simulink model "combining_trajectory_parking_pietro"  (R2025b)
settings: Solver=ode5  StartTime=0.0  StopTime=25  FixedStep=0.0001  MaxStep=0.01  RelTol=1e-3
values from neighbouring files (symbols this model uses):
  ang_velocity = 3    [traj.m]
  speed = 15    [traj.m]
  time_vec_circ = time_vec_circ'    [traj.m]
  waypoints = [ ... (first row only)    [traj.m]
libraries: dspsigops x3
settings Model: Creator=Cris  LastModifiedBy=pietr
settings DebuggingCC: UnderspecifiedInitializationDetection=Classic  MergeDetectMultiDrivingBlocksExec=none
settings ModelReferenceCC: PropagateSignalLabelsOutOfModel=off

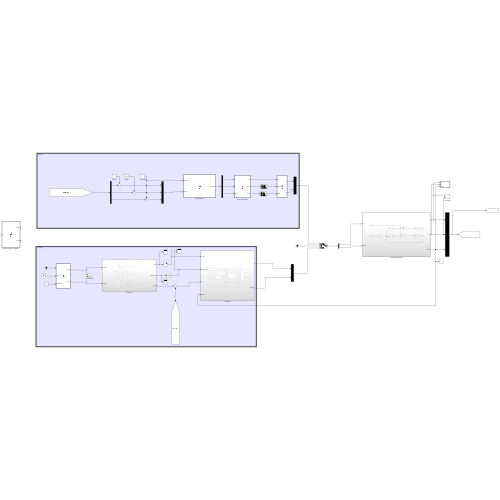
[thumbnail: Simulink's stored preview of the top-level diagram]
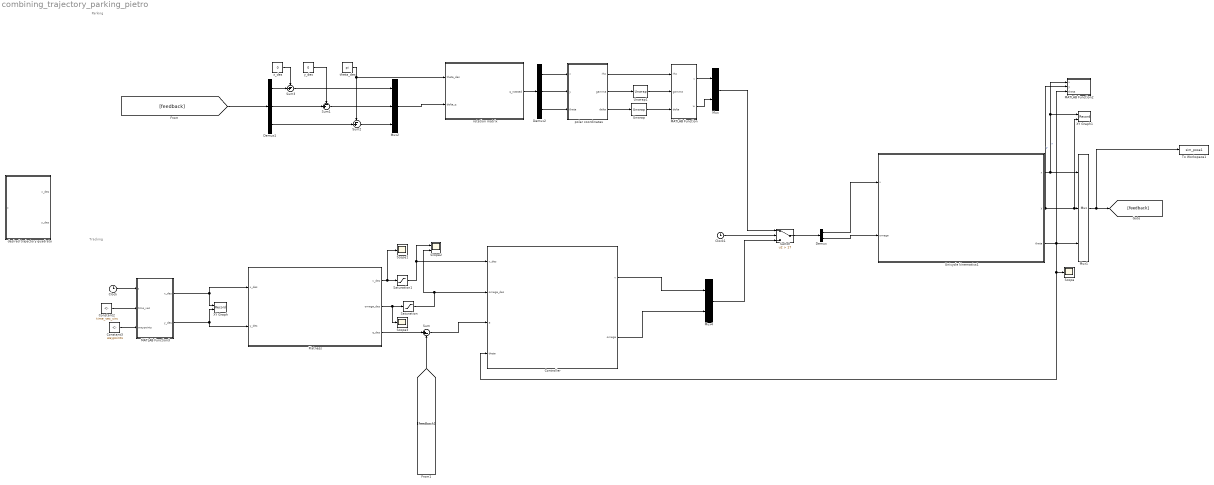
== system combining_trajectory_parking_pietro ==
  note: Tracking
  note: Parking
  Clock : Clock
  Clock1 : Clock
  Constant2 : Constant  Value=time_vec_circ
  Constant3 : Constant  Value=waypoints
  Controller : Subsystem
  Demux : Demux  Outputs=2
  Demux1 : Demux  Outputs=3
  Demux2 : Demux  Outputs=3
  Flatness : Subsystem
  MATLAB Function : MATLAB Function  TreatAsAtomicUnit=on
  MATLAB Function2 : MATLAB Function  TreatAsAtomicUnit=on
  MATLAB Function3 : MATLAB Function  TreatAsAtomicUnit=on
  Mux : Mux  Inputs=2
  Mux1 : Mux  Inputs=3
  Mux2 : Mux  Inputs=3
  Mux4 : Mux  Inputs=2
  Saturation : Saturate  UpperLimit=ang_velocity  LowerLimit=-ang_velocity
  Saturation1 : Saturate  UpperLimit=speed  LowerLimit=-speed
  Scope : Scope
      settings: ActiveDisplayYMinimum=-2.2678628072381004  ActiveDisplayYMaximum=10.713846589075981
  Scope1 : Scope
      settings: ActiveDisplayYMinimum=-58.541647894510909  ActiveDisplayYMaximum=33.790255014407059  DataLoggingVariableName=ScopeData3
  Scope2 : Scope  NumInputPorts=2
      settings: ActiveDisplayYMinimum=0.14603727460674376  ActiveDisplayYMaximum=5.9509475084943659
  Scope3 : Scope
      settings: ActiveDisplayYMinimum=-7.9417132034456789E+8  ActiveDisplayYMaximum=7.1473011331260653E+9  DataLoggingVariableName=ScopeData4
  Sum : Sum  Inputs=|+-
  Sum1 : Sum  Inputs=-+|
  Sum2 : Sum  Inputs=-+|
  Sum3 : Sum  Inputs=-+|
  Switch : Switch  Criteria=u2 > Threshold  Threshold=17  SaturateOnIntegerOverflow=off  InputSameDT=off
  To Workspace1 : ToWorkspace  VariableName=sim_pose1  SaveFormat=Timeseries  SampleTime=-1
  Unicycle kinematics1 : Subsystem
  Unwrap : dspsigops/Unwrap  tol=pi  InputProcessing=Columns as channels (frame based)  running=off
  Unwrap1 : dspsigops/Unwrap  tol=pi  InputProcessing=Columns as channels (frame based)  running=off
  XY Graph : Record  NumPorts=2.0  FileSettingsInternal="{\"entries\":[{\"content\":{\"excelSettings\":{\"content\":{},\"type\":\"Streamout.ExcelSettings\"},\"parquetSettings\":{\"content\":{},\"type\":\"Streamout.ParquetSettings\"}},\"type\":\"Streamout.FileSettingStorage\",\"uuid\":\"\"}],\"packageUris\":[\"http:\\/\\/schema.mathworks.com\\/mf0\\/streamout_blocks\\/R2020a\"],\"version\":\"1.0\"}"  FrameSettings=[0, 0]  Layout=[1 1]  SignalsInternal="{\"entries\":[{\"content\":{\"signals\":[{\"content\":{\"blockPath\":[],\"dimensions\":[1],\"domain\":\"\",\"lineColor\":\"#a2142f\",\"plots\":[ 1 ],\"port\":1,\"sid\":[\"\"],\"signalID\":1,\"signalName\":\"MATLAB Function3:1\"},\"type\":\"RecordBlkView.Signal\",\"uuid\":\"\"},{\"content\":{\"blockPath\":[],\"dimensions\":[1],\"domain\":\"\",\"lineColor\":\"#139fff\",\"plots\":[ 1 ],\"port\":2,\"sid\":[\"\"],\"signalID\":2,\"signalName\":\"MATLAB Function3:2\"},\"type\":\"RecordBlkView.Signal\",\"uuid\":\"\"}]},\"type\":\"RecordBlkView.InputSignals\",\"uuid\":\"\"}],\"packageUris\":[\"http:\\/\\/schema.mathworks.com\\/mf0\\/streamout_blocks\\/R2020a\"],\"version\":\"1.0\"}"  VisualizationBindings="{\"xyplotplugin\":{\"info\":[{\"series\":[{\"bindingParametersList\":[{\"parameter\":\"X-Axis\",\"signalID\":1,\"signalName\":\"MATLAB Function3:1\"},{\"parameter\":\"Y-Axis\",\"signalID\":2,\"signalName\":\"MATLAB Function3:2\"}],\"seriesID\":0}],\"subplotID\":1}]}}"  CompatibilityTag=XY
  XY Graph1 : Record  NumPorts=2.0  FileSettingsInternal="{\"entries\":[{\"content\":{\"excelSettings\":{\"content\":{},\"type\":\"Streamout.ExcelSettings\"},\"parquetSettings\":{\"content\":{},\"type\":\"Streamout.ParquetSettings\"}},\"type\":\"Streamout.FileSettingStorage\",\"uuid\":\"\"}],\"packageUris\":[\"http:\\/\\/schema.mathworks.com\\/mf0\\/streamout_blocks\\/R2020a\"],\"version\":\"1.0\"}"  FrameSettings=[0, 0]  Layout=[1 1]  SignalsInternal="{\"entries\":[{\"content\":{\"signals\":[{\"content\":{\"blockPath\":[],\"dimensions\":[1],\"domain\":\"\",\"lineColor\":\"#a2142f\",\"plots\":[ 1 ],\"port\":1,\"sid\":[\"\"],\"signalID\":1,\"signalName\":\"x\"},\"type\":\"RecordBlkView.Signal\",\"uuid\":\"\"},{\"content\":{\"blockPath\":[],\"dimensions\":[1],\"domain\":\"\",\"lineColor\":\"#139fff\",\"plots\":[ 1 ],\"port\":2,\"sid\":[\"\"],\"signalID\":2,\"signalName\":\"y\"},\"type\":\"RecordBlkView.Signal\",\"uuid\":\"\"}]},\"type\":\"RecordBlkView.InputSignals\",\"uuid\":\"\"}],\"packageUris\":[\"http:\\/\\/schema.mathworks.com\\/mf0\\/streamout_blocks\\/R2020a\"],\"version\":\"1.0\"}"  VisualizationBindings="{\"xyplotplugin\":{\"info\":[{\"series\":[{\"bindingParametersList\":[{\"parameter\":\"X-Axis\",\"signalID\":1,\"signalName\":\"x\"},{\"parameter\":\"Y-Axis\",\"signalID\":2,\"signalName\":\"y\"}],\"seriesID\":0}],\"subplotID\":1}]}}"  CompatibilityTag=XY
  desired trajectory quadrato : MATLAB Function  TreatAsAtomicUnit=on
  polar coordinates : MATLAB Function  TreatAsAtomicUnit=on
  rotation matrix : MATLAB Function  TreatAsAtomicUnit=on
  theta_des : Constant  Value=pi
  x_des : Constant  Value=0
  y_des : Constant  Value=0
  wires:
  Flatness/3(q_des) -> Sum/1
  Controller/2(omega) -> Mux4/2
  Demux1/3 -> Sum2/2
  theta_des/1 -> Sum2/1, rotation matrix/1(theta_des)
  rotation matrix/1(q_rotated) -> Demux2/1
  Sum1/1 -> Mux2/2
  Unwrap/1 -> MATLAB Function/3(delta)
  Sum2/1 -> Mux2/3
  y_des/1 -> Sum1/1
  x_des/1 -> Sum3/1
  Demux2/1 -> polar coordinates/1(x)
  Mux1/1 -> [feedback], To Workspace1/1
  Mux2/1 -> rotation matrix/2(delta_q)
  Demux2/3 -> polar coordinates/3(theta)
  Unicycle kinematics1/2(y) -> MATLAB Function2/2(y), XY Graph1/2, Mux1/2  "y"
  Unicycle kinematics1/1(x) -> MATLAB Function2/1(x), XY Graph1/1, Mux1/1  "x"
  Unwrap1/1 -> MATLAB Function/2(gamma)
  Sum3/1 -> Mux2/1
  Unicycle kinematics1/3(theta) -> Controller/4(theta), Scope/1, Mux1/3, MATLAB Function2/3(theta)
  polar coordinates/3(delta) -> Unwrap/1
  polar coordinates/2(gamma) -> Unwrap1/1
  Demux1/2 -> Sum1/2
  Demux1/1 -> Sum3/2
  Demux2/2 -> polar coordinates/2(y)
  polar coordinates/1(rho) -> MATLAB Function/1(rho)
  Clock1/1 -> Switch/2
  [feedback] -> Demux1/1
  [feedback] -> Sum/2
  MATLAB Function/1(v) -> Mux/1
  MATLAB Function/2(w) -> Mux/2
  Demux/1 -> Unicycle kinematics1/1(v)
  Demux/2 -> Unicycle kinematics1/2(omega)
  Controller/1(v) -> Mux4/1
  Mux/1 -> Switch/1
  Switch/1 -> Demux/1
  Mux4/1 -> Switch/3
  Constant3/1 -> MATLAB Function3/3(waypoints)
  MATLAB Function3/1(x_des) -> Flatness/1(x_des), XY Graph/1
  MATLAB Function3/2(y_des) -> XY Graph/2, Flatness/2(y_des)
  Flatness/2(omega_des) -> Scope3/1, Saturation/1
  Saturation/1 -> Scope2/2, Controller/2(omega_des)
  Flatness/1(v_des) -> Saturation1/1, Scope1/1
  Saturation1/1 -> Controller/1(v_des), Scope2/1
  Sum/1 -> Controller/3(e)
  Clock/1 -> MATLAB Function3/1(t)
  Constant2/1 -> MATLAB Function3/2(time_vec)

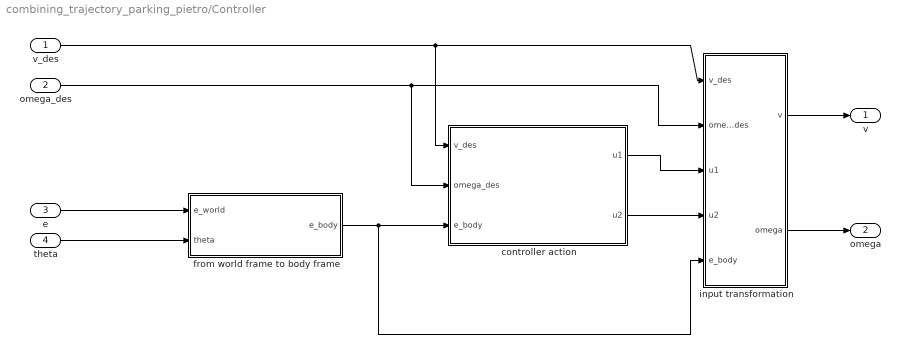
== system combining_trajectory_parking_pietro/Controller ==
  v_des : Inport
  omega_des : Inport  Port=2
  e : Inport  Port=3
  theta : Inport  Port=4
  controller action : MATLAB Function  TreatAsAtomicUnit=on
  from world frame to body frame : MATLAB Function  TreatAsAtomicUnit=on
  input transformation : MATLAB Function  TreatAsAtomicUnit=on
  v : Outport
  omega : Outport  Port=2
  wires:
  e/1 -> from world frame to body frame/1(e_world)
  theta/1 -> from world frame to body frame/2(theta)
  from world frame to body frame/1(e_body) -> input transformation/5(e_body), controller action/3(e_body)
  v_des/1 -> controller action/1(v_des), input transformation/1(v_des)
  controller action/2(u2) -> input transformation/4(u2)
  input transformation/2(omega) -> omega/1
  input transformation/1(v) -> v/1
  omega_des/1 -> input transformation/2(omega_des), controller action/2(omega_des)
  controller action/1(u1) -> input transformation/3(u1)

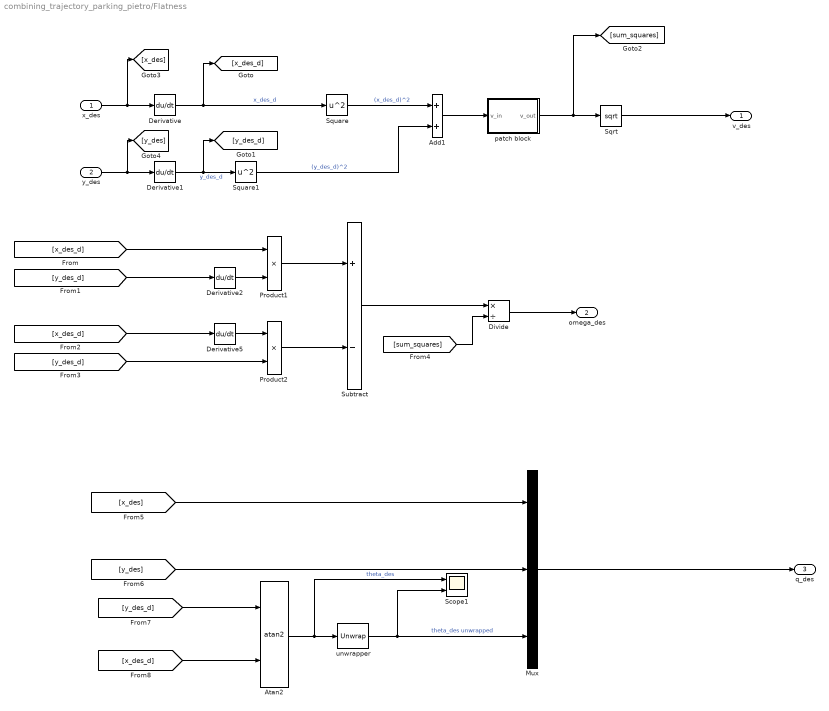
== system combining_trajectory_parking_pietro/Flatness ==
  x_des : Inport
  y_des : Inport  Port=2
  Add1 : Sum
  Atan2 : Trigonometry  Operator=atan2
  Derivative{,1..2,5} (4 alike) : Derivative
  Divide : Product  Inputs=*/
  Mux : Mux  Inputs=3
  Product1 : Product
  Product2 : Product
  Scope1 : Scope  NumInputPorts=2
      settings: ActiveDisplayYMinimum=-16.66586404144536  ActiveDisplayYMaximum=10.473474164834791  DataLoggingVariableName=ScopeData2  DataLoggingSaveFormat=Array
  Sqrt : Sqrt
  Square : Math  Operator=square
  Square1 : Math  Operator=square
  Subtract : Sum  Inputs=+-
  patch block : MATLAB Function  TreatAsAtomicUnit=on
  unwrapper : dspsigops/Unwrap  tol=pi  InputProcessing=Columns as channels (frame based)  running=off
  v_des : Outport
  omega_des : Outport  Port=2
  q_des : Outport  Port=3
  wires:
  x_des/1 -> [x_des], Derivative/1
  y_des/1 -> [y_des], Derivative1/1
  Derivative/1 -> [x_des_d], Square/1  "x_des_d"
  Derivative1/1 -> [y_des_d], Square1/1  "y_des_d"
  Square/1 -> Add1/1  "(x_des_d)^2"
  Square1/1 -> Add1/2  "(y_des_d)^2"
  [x_des_d] -> Product1/1
  [y_des_d] -> Derivative2/1
  Derivative2/1 -> Product1/2
  [y_des_d] -> Product2/2
  [x_des_d] -> Derivative5/1
  Derivative5/1 -> Product2/1
  Product1/1 -> Subtract/1
  Product2/1 -> Subtract/2
  Subtract/1 -> Divide/1
  [sum_squares] -> Divide/2
  Divide/1 -> omega_des/1
  Mux/1 -> q_des/1
  Atan2/1 -> unwrapper/1, Scope1/1  "theta_des"
  [x_des_d] -> Atan2/2
  [y_des_d] -> Atan2/1
  Add1/1 -> patch block/1(v_in)
  patch block/1(v_out) -> [sum_squares], Sqrt/1
  Sqrt/1 -> v_des/1
  [x_des] -> Mux/1
  [y_des] -> Mux/2
  unwrapper/1 -> Mux/3, Scope1/2  "theta_des unwrapped"

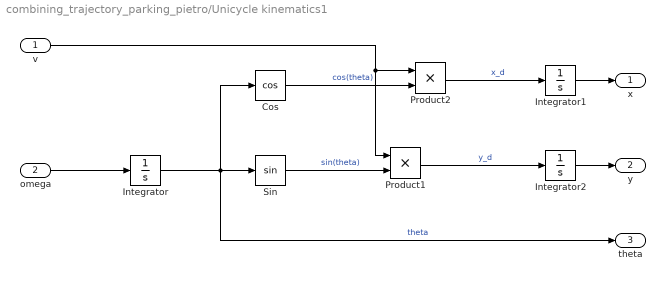
== system combining_trajectory_parking_pietro/Unicycle kinematics1 ==
  v : Inport
  omega : Inport  Port=2
  Cos : Trigonometry  Operator=cos
  Integrator : Integrator  InitialCondition=pi
  Integrator1 : Integrator  InitialCondition=10
  Integrator2 : Integrator
  Product1 : Product
  Product2 : Product
  Sin : Trigonometry
  x : Outport
  y : Outport  Port=2
  theta : Outport  Port=3
  wires:
  omega/1 -> Integrator/1
  Integrator/1 -> theta/1, Cos/1, Sin/1  "theta"
  Cos/1 -> Product2/2  "cos(theta)"
  Sin/1 -> Product1/2  "sin(theta)"
  v/1 -> Product2/1, Product1/1
  Integrator1/1 -> x/1
  Product2/1 -> Integrator1/1  "x_d"
  Integrator2/1 -> y/1
  Product1/1 -> Integrator2/1  "y_d"

== matlab function combining_trajectory_parking_pietro/Controller/controller action ==
  data: v_des input; omega_des input; e_body input; u1 output; u2 output
function [u1, u2] = fcn(v_des, omega_des, e_body)

% TO DO: parametri da modfiicare
d = 1/sqrt(2);
a = 10; %10;



% parametri controllore
k1 = 2*d*a;

% if abs(v_des) < 1e-4
%     if v_des >= 0
%         v_des = 1e-4;
%     else
%         v_des = -1e-4;
%     end
% end

k3 = k1;
k2 = ( a^2-(omega_des)^2 ) / v_des;

u1 = [-k1, 0, 0] * e_body;
u2 = [0, -k2, -k3] * e_body;

== matlab function combining_trajectory_parking_pietro/Controller/from world frame to body frame ==
  data: e_world input; e_body output size=3; theta input
function e_body = fcn(e_world, theta)


% Transformation matrix
R = [cos(theta), sin(theta), 0; 
    -sin(theta), cos(theta), 0;
    0, 0, 1];

% get error in body frame
e_body = R*e_world;

== matlab function combining_trajectory_parking_pietro/Controller/input transformation ==
  data: v_des input; v output size=1; omega_des input; u1 input; u2 input; e_body input size=3; omega output
function [v, omega] = fcn(v_des, omega_des, u1, u2, e_body)


v = v_des * cos(e_body(3)) - u1;
omega = omega_des - u2;

== matlab function combining_trajectory_parking_pietro/rotation matrix ==
  data: theta_des input; delta_q input; q_rotated output
function q_rotated  = fcn(theta_des, delta_q)

% rotation matrix
R = [cos(theta_des), sin(theta_des), 0;
    -sin(theta_des), cos(theta_des), 0; 
    0,              0,              1];

% rotate
q_rotated = R*delta_q;

== matlab function combining_trajectory_parking_pietro/Flatness/patch block ==
  data: v_in input size=1; v_out output size=1
function v_out = fcn(v_in)

if abs(v_in) < 1e-4
    if v_in >= 0
        v_in = 1e-4;
    else
        v_in = -1e-4;
    end
end
v_out = v_in;

== matlab function combining_trajectory_parking_pietro/desired trajectory quadrato ==
  data: t input; x_des output; y_des output
function [x_des, y_des] = fcn(t)

% % configurable:
% radius = 5;
% omega_des = 0.2;
% 
% % desired trajectory
% x_des = -radius*cos(omega_des*t);
% y_des = -radius*sin(omega_des*t);


% % configurable:
% radius = 10;
% omega_des = 0.5;
% 
% % desired trajectory
% x_des = radius*cos(omega_des*t);
% y_des = radius*sin(omega_des*t);
% 


if t <= 10
    x_des = 10+t;
    y_des = 10;
elseif  t <= 20
    x_des = 20;
    y_des = 0+t;
elseif  t <= 30
    x_des = 40-t;
    y_des = 20;
elseif  t <= 40
    x_des = 10;
    y_des = 50-t;
else
    x_des = 100;
    y_des = 100;
end

== matlab function combining_trajectory_parking_pietro/MATLAB Function ==
  data: v output; rho input; gamma input; w output; delta input
function [v , w] = fcn(rho, gamma, delta)

% adjust gains
k1 = 3;%3
k2 = 6;%6
k3 = 1.5;%1.5


% controller

v = k1*rho*cos(gamma);

if (abs(gamma) > 0.001)
    temp = sin(gamma)/gamma;
else
    temp = 1;
end

w = k2*gamma + (k1*temp*cos(gamma))*(gamma+k3*delta);

if rho < 0.01
    v = 0;
    w = 0;
end

== matlab function combining_trajectory_parking_pietro/MATLAB Function2 ==
  settings: updateMethod=DISCRETE
  data: x input; y input; theta input
function Animazione_Mappa(x, y, theta)
    % Dichiara la funzione come esterna a Simulink
    coder.extrinsic('real_time_traj');
    
    % Passa i dati alla funzione MATLAB standard
    real_time_traj(x, y, theta);
end

== matlab function combining_trajectory_parking_pietro/MATLAB Function3 ==
  data: t input; x_des output; time_vec input; waypoints input; y_des output
function [x_des, y_des] = fcn(t, time_vec, waypoints)

    t_start_circle = time_vec(8);
    t_end_circle = time_vec(9);

    if t <= t_start_circle

        t_1 = time_vec(1:8);
        traj_x_1 = waypoints(1:8, 1);
        traj_y_1 = waypoints(1:8, 2);

        x_des = interp1(t_1, traj_x_1, t, 'pchip');
        y_des = interp1(t_1, traj_y_1, t, 'pchip');

    elseif t > t_start_circle && t <= t_end_circle

        circle_start = waypoints(8,:);
        circle_end = waypoints(9,:);

        centre = [(circle_start(1) + circle_end(1))/2, (circle_start(2) + circle_end(2))/2];

        radius = norm(circle_start - circle_end) / 2;

        start_ang = atan2(circle_start(2) - centre(2), circle_start(1) - centre(1));
        stop_ang = atan2(circle_end(2) - centre(2), circle_end(1) - centre(1));

        angles = [start_ang, stop_ang];

        theta = interp1([t_start_circle, t_end_circle], angles, t, 'pchip');

        x_des = centre(1) + radius * cos(theta);
        y_des = centre(2) + radius * sin(theta);

    else

        t_2 = time_vec(9:12);
        traj_x_2 = waypoints(9:12, 1);
        traj_y_2 = waypoints(9:12, 2);

        t_end = time_vec(12);

        if t < t_end
            x_des = interp1(t_2, traj_x_2, t, 'pchip');
            y_des = interp1(t_2, traj_y_2, t, 'pchip');
        else
            x_des = waypoints(12,1);
            y_des = waypoints(12,2);
    end

end

== matlab function combining_trajectory_parking_pietro/polar coordinates ==
  data: x input; rho output; gamma output; delta output; y input; theta input
function [rho, gamma, delta] = fcn(x, y, theta)

rho = sqrt(x^2+y^2);
gamma = atan2(y, x) + pi - theta;
delta = gamma + theta;
